simulink model "GaitGeneration"  (R2026a)
settings: Solver=FixedStepAuto  StopTime=10  FixedStep=0.001
values from neighbouring files (symbols this model uses):
  db = database()    [LeggedRobotSim.m]    (also in dbFunc.m; parameterSweep.m; parameterSweepDims.m)
libraries: simulink x2
settings Model: Creator=indyg  LastModifiedBy=indyg

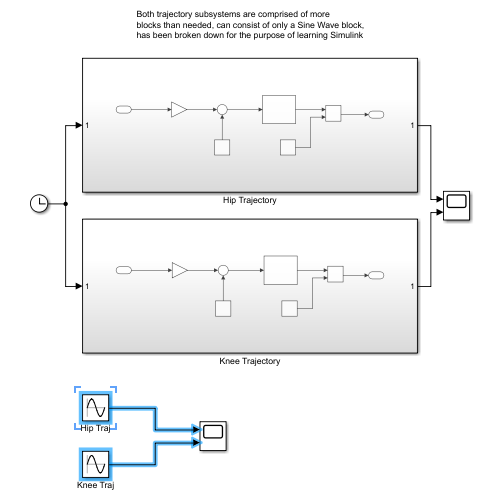
[thumbnail: Simulink's stored preview of the top-level diagram]
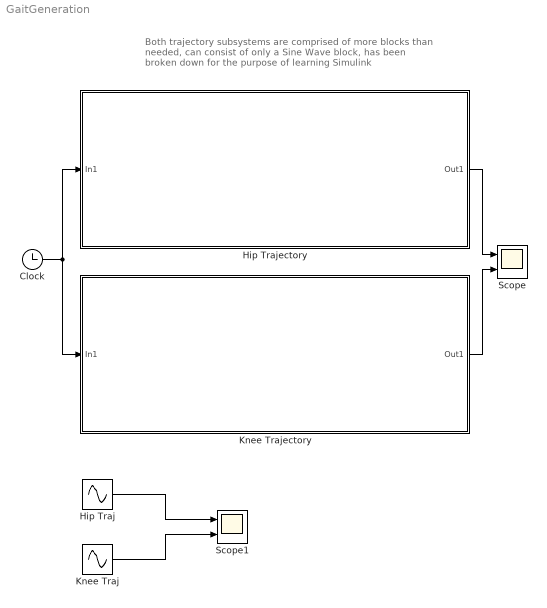
== system GaitGeneration ==
  note: Both trajectory subsystems are comprised of more
      | blocks than needed, can consist of only a Sine Wave block,
      | has been broken down for the purpose of learning Simulink
  Clock : Clock
  Hip Traj : Sin  Amplitude=db.gait.theta_amp(1)  Frequency=db.gait.f_hip*pi*2  Phase=db.gait.phi_hip  SampleTime=0
  Hip Trajectory : Subsystem
  Knee Traj : Sin  Amplitude=db.gait.theta_amp(2)  Frequency=db.gait.f_knee*pi*2  Phase=db.gait.phi_knee  SampleTime=0
  Knee Trajectory : Subsystem
  Scope : Scope  NumInputPorts=2
      settings: ActiveDisplayYMinimum=-0.97928494602875948  ActiveDisplayYMaximum=0.98115448511399517
  Scope1 : Scope  NumInputPorts=2
  wires:
  Clock/1 -> Knee Trajectory/1(In1), Hip Trajectory/1(In1)
  Hip Trajectory/1(Out1) -> Scope/1
  Knee Trajectory/1(Out1) -> Scope/2
  Hip Traj/1 -> Scope1/1
  Knee Traj/1 -> Scope1/2

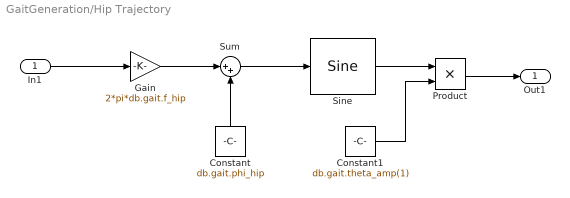
== system GaitGeneration/Hip Trajectory ==
  In1 : Inport
  Constant : Constant  Value=db.gait.phi_hip
  Constant1 : Constant  Value=db.gait.theta_amp(1)
  Gain : Gain  Gain=2*pi*db.gait.f_hip
  Product : Product
  Sine : simulink/Lookup Tables/Sine  Formula=sin(2*pi*u)  NumDataPoints=(2^5)+1  OutputWordLength=16  InternalRulePriority=Speed
  Sum : Sum  Inputs=|++
  Out1 : Outport
  wires:
  Sum/1 -> Sine/1
  Constant/1 -> Sum/2
  Product/1 -> Out1/1
  Constant1/1 -> Product/2
  In1/1 -> Gain/1
  Gain/1 -> Sum/1
  Sine/1 -> Product/1

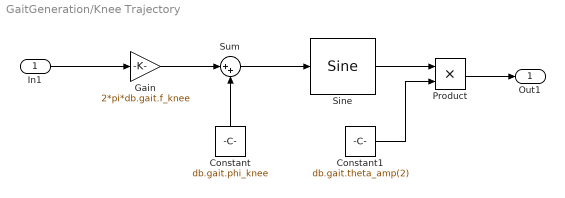
== system GaitGeneration/Knee Trajectory ==
  In1 : Inport
  Constant : Constant  Value=db.gait.phi_knee
  Constant1 : Constant  Value=db.gait.theta_amp(2)
  Gain : Gain  Gain=2*pi*db.gait.f_knee
  Product : Product
  Sine : simulink/Lookup Tables/Sine  Formula=sin(2*pi*u)  NumDataPoints=(2^5)+1  OutputWordLength=16  InternalRulePriority=Speed
  Sum : Sum  Inputs=|++
  Out1 : Outport
  wires:
  Sum/1 -> Sine/1
  Constant/1 -> Sum/2
  Product/1 -> Out1/1
  Constant1/1 -> Product/2
  In1/1 -> Gain/1
  Gain/1 -> Sum/1
  Sine/1 -> Product/1
